simulink model "bicycle_drift_model_drive_force"  (R2016a)
settings: Solver=VariableStepAuto  StartTime=0.0  StopTime=200  MaxStep=1e-3  RelTol=1e-3
values from neighbouring files (symbols this model uses):
  a = 0.1329    [dynamics.m]    (also in setup.m; tire_test.m = 0.11372)
  b = 0.1221    [dynamics.m]    (also in setup.m; tire_test.m = 0.14328)
  C_alpha = 120000    [dynamics.m]    (also in setup.m; tire_test.m = 197)
  initial_states = [0 0 0.1]    [setup.m]
  Iz = 0.020899525    [dynamics.m]    (also in setup.m; tire_test.m = 0.025)
  L = 0.255    [dynamics.m]    (also in setup.m; tire_test.m = 0.257; veh_object2.m = obj_length)
  m = 2.622    [dynamics.m]    (also in setup.m; tire_test.m = 2.35)
  mu = 0.37    [dynamics.m]    (also in setup.m; tire_test.m = 1.31)
undefined symbols (not defined in the file): animation_update_interval, datetime, enable_CG_trace, enable_rearAxle_trace, plotAxisLimitMode, plotAxisLimits, save_anim_frames, vehicle_length, vehicle_width
libraries: simulink x2, vrlib x1
settings Model: Creator=Cyrus  LastModifiedBy=Cyrus

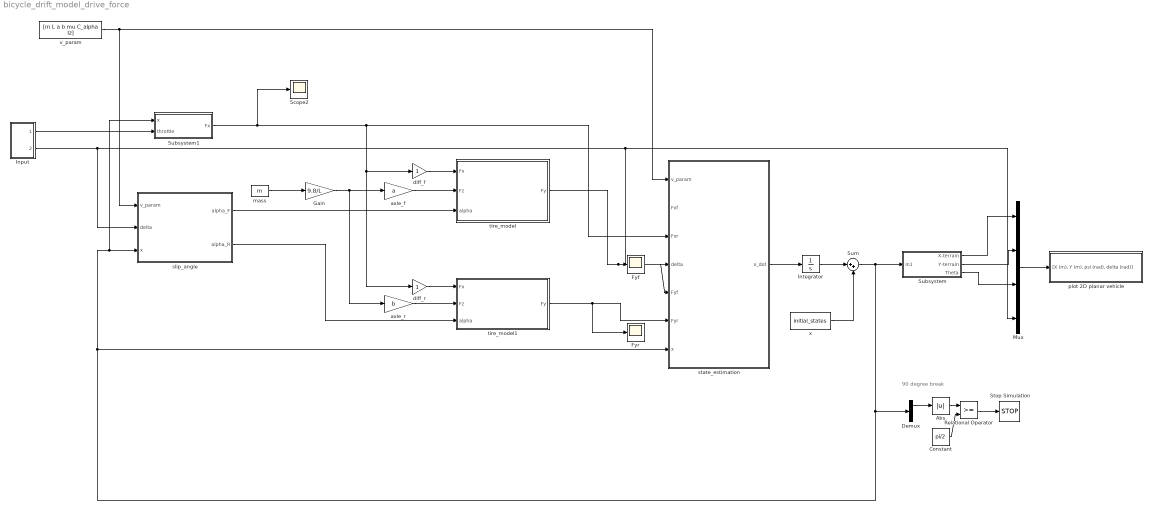
== system bicycle_drift_model_drive_force ==
  note: 90 degree break
  Abs : Abs
  Constant : Constant  Value=pi/2
  Demux : Demux  Outputs=3
  Fyf : Scope
  Fyr : Scope
  Gain : Gain  Gain=9.8/L
  Input : Subsystem
  Integrator : Integrator
  Mux : Mux
  Relational Operator : RelationalOperator  OutDataTypeStr=boolean
  Scope2 : Scope
  Stop Simulation : Stop
  Subsystem : Subsystem
  Subsystem1 : Subsystem
  Sum : Sum  Inputs=|++
  axle_f : Gain  Gain=a
  axle_r : Gain  Gain=b
  diff_f : Gain
  diff_r : Gain
  mass : Constant  Value=m
  plot 2D planar vehicle : Subsystem  mask(6DoF Animation){axisMode=plotAxisLimitMode, ax=plotAxisLimits, Ts=animation_update_interval, enable_CG_trace=enable_CG_trace, enable_rearAxle_trace=enable_rearAxle_trace, save_anim_frames=save_anim_frames, anim_frame_name_str=char(datetime('now','Format','yyyy-MM-dd_HH_mm_ss')), L=vehicle_length, W=vehicle_width}
      mask prompts: axisMode "Axis Mode (0->auto, 1->fixed, BOTH use Axes Limits below)"; ax "Axes limits [xmin xmax ymin ymax] (m):"; Ts "Time interval between updates (s):"; enable_CG_trace "Enable vehicle CG trace? (0/1)"; enable_rearAxle_trace "Enable rear axle trace? (0/1)"; save_anim_frames "Save animaton frames? (0/1)"; anim_frame_name_str "Animation sequence name (if save frames==1)"; L "Vehicle length (m)"; W "Vehicle width (m)"
      mask help:
      | Create a 2D animated view of a steering vehicle model with tires.
      |
      | Marc Compere
      | CompereM@saic.com
      | created : 22 August 2002
      | modified: 28 Dec 2015
      mask init:
      | Config.axisMode=axisMode;
      | Config.ax=ax;
      | Config.Ts=Ts;
      | Config.enable_CG_trace=enable_CG_trace;
      | Config.enable_rearAxle_trace=enable_rearAxle_trace;
      | Config.save_anim_frames=save_anim_frames;
      | Config.anim_frame_name_str=anim_frame_name_str;
      | Config.L=L;
      | Config.W=W;
      mask Help:
      | <p>This block generates a 3 dimensional display of a simulation trajectory, with the craft orientation displayed during flight</p>
      | 
      | <p>There are two inputs to this block, Position and Euler.  These inputs contain more than one signal as described below.</p>
      | 
      | <p><H4>Block Vector Input - Position</H4>
      | <ul>
      | <li>X Position</li>
      | <li>Y Position</li>
      | <li>Z Position</li>
      | </ul>
      | </p>
      | 
      | <p><H4>Block Vector Input - Euler</H4>
      |     <ul>
      |     <li>Roll Attitude</li>
      |     <li>Pitch Attitude</li>
      |     <li>Yaw Attitude</li>
      |    </ul>
      |    </p>
  slip_angle : MATLAB Function  TreatAsAtomicUnit=on
  state_estimation : MATLAB Function  TreatAsAtomicUnit=on
  tire_model : Subsystem
  tire_model1 : Subsystem
  v_param : Constant  Value=[m L a b mu C_alpha Iz]
  x : Constant  Value=initial_states
  wires:
  mass/1 -> Gain/1
  axle_f/1 -> tire_model/2(Fz)
  axle_r/1 -> tire_model1/2(Fz)
  slip_angle/1(alpha_F) -> tire_model/3(alpha)
  Gain/1 -> axle_r/1, axle_f/1
  Sum/1 -> slip_angle/3(x), Subsystem1/1(x), state_estimation/7(x), Demux/1, Subsystem/1(In1)
  state_estimation/1(x_dot) -> Integrator/1
  tire_model/1(Fy) -> Fyf/1, state_estimation/5(Fyf)
  tire_model1/1(Fy) -> Fyr/1, state_estimation/6(Fyr)
  Input/1(Throttle) -> Subsystem1/2(throttle)
  Integrator/1 -> Sum/1
  x/1 -> Sum/2
  Subsystem/1(X-terrain) -> Mux/1
  Subsystem/2(Y-terrain) -> Mux/2
  Subsystem/3("Theta ") -> Mux/3
  Mux/1 -> plot 2D planar vehicle/1("[X (m), Y (m), psi (rad), delta (rad)]")
  v_param/1 -> state_estimation/1(v_param), slip_angle/1(v_param)
  slip_angle/2(alpha_R) -> tire_model1/3(alpha)
  Input/2(Steering) -> Mux/4, state_estimation/4(delta), slip_angle/2(delta)
  diff_f/1 -> tire_model/1(Fx)
  Subsystem1/1(Fx) -> diff_f/1, diff_r/1, state_estimation/3(Fxr), Scope2/1
  diff_r/1 -> tire_model1/1(Fx)
  Demux/1 -> Abs/1
  Abs/1 -> Relational Operator/1
  Constant/1 -> Relational Operator/2
  Relational Operator/1 -> Stop Simulation/1

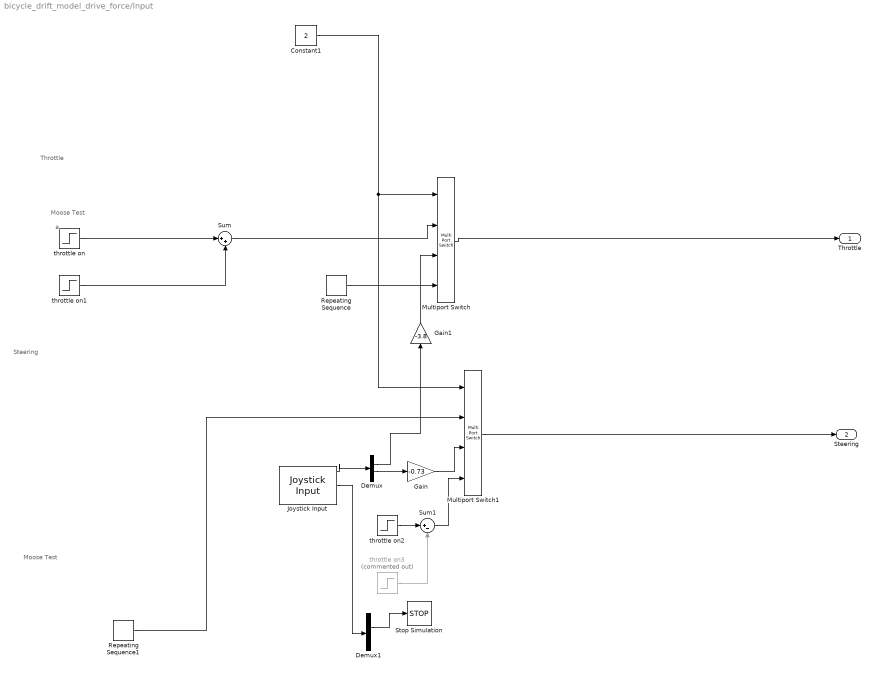
== system bicycle_drift_model_drive_force/Input ==
  note: a
  note: Steering
  note: Throttle
  note: Moose Test
  note: Moose Test
  Constant1 : Constant  Value=2
  Demux : Demux
  Demux1 : Demux  Outputs=12
  Gain : Gain  Gain=-0.73
  Gain1 : Gain  Gain=-3.8  OutMin=[0.1]
  Joystick Input : vrlib/Joystick Input  joyid=1  adjustports=on  forcefeed=off
  Multiport Switch : MultiPortSwitch
  Multiport Switch1 : MultiPortSwitch
  Repeating Sequence : simulink/Sources/Repeating Sequence  rep_seq_t=[0 2 2.1 2.5 2.6 200]  rep_seq_y=[1 1 -3.5 -3.5 0 0]
  Repeating Sequence1 : simulink/Sources/Repeating Sequence  rep_seq_t=[0 0.2 0.4 0.5 0.7 1.4 1.6 2 2.2 2.3 2.7 200]  rep_seq_y=[0 0 0.8 0.8 -0.8 -0.8 0.8 0.8 -0.8 -0.8 0 0]
  Stop Simulation : Stop
  Sum : Sum  Inputs=|++
  Sum1 : Sum  Inputs=|+-
  throttle on : Step  Time=0.2  After=2.7  SampleTime=0
  throttle on1 : Step  Time=2  After=-2.7  SampleTime=0
  throttle on2 : Step  Time=0  After=0.5  SampleTime=0
  throttle on3 : Step  Commented=on  Time=2  After=-0.8  SampleTime=0
  Throttle : Outport
  Steering : Outport  Port=2
  wires:
  Multiport Switch1/1 -> Steering/1
  Sum/1 -> Multiport Switch/2
  throttle on1/1 -> Sum/2
  throttle on/1 -> Sum/1
  Gain/1 -> Multiport Switch1/3
  Demux/3 -> Gain/1
  Joystick Input/1 -> Demux/1
  Gain1/1 -> Multiport Switch/3
  Constant1/1 -> Multiport Switch1/1, Multiport Switch/1
  Demux/2 -> Gain1/1
  Repeating Sequence/1 -> Multiport Switch/4
  Multiport Switch/1 -> Throttle/1
  throttle on2/1 -> Sum1/1
  Sum1/1 -> Multiport Switch1/4
  throttle on3/1 -> Sum1/2
  Repeating Sequence1/1 -> Multiport Switch1/2
  Joystick Input/2 -> Demux1/1
  Demux1/5 -> Stop Simulation/1

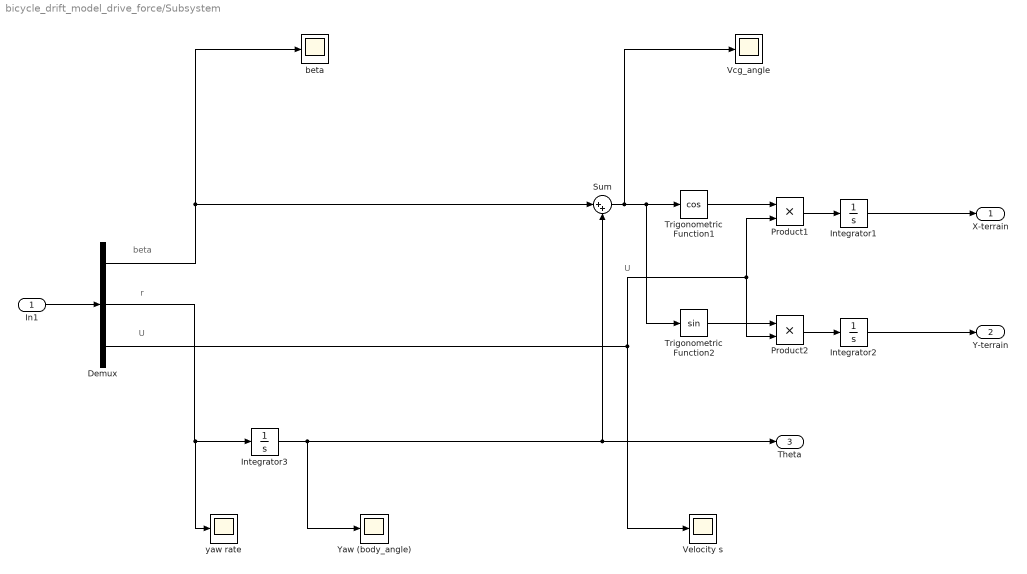
== system bicycle_drift_model_drive_force/Subsystem ==
  note: r
  note: U
  note: U
  note: beta
  In1 : Inport
  Demux : Demux  Outputs=3
  Integrator1 : Integrator
  Integrator2 : Integrator
  Integrator3 : Integrator
  Product1 : Product
  Product2 : Product
  Sum : Sum  Inputs=|++
  Trigonometric Function1 : Trigonometry  Operator=cos
  Trigonometric Function2 : Trigonometry
  Vcg_angle : Scope
  Velocity s : Scope
  Yaw (body_angle) : Scope
  beta : Scope
  yaw rate : Scope
  X-terrain : Outport
  Y-terrain : Outport  Port=2
  "Theta " : Outport  Port=3
  wires:
  In1/1 -> Demux/1
  Demux/2 -> yaw rate/1, Integrator3/1
  Demux/1 -> Sum/1, beta/1
  Trigonometric Function1/1 -> Product1/1
  Trigonometric Function2/1 -> Product2/1
  Product1/1 -> Integrator1/1
  Product2/1 -> Integrator2/1
  Integrator1/1 -> X-terrain/1
  Integrator2/1 -> Y-terrain/1
  Integrator3/1 -> "Theta "/1, Sum/2, Yaw (body_angle)/1
  Sum/1 -> Vcg_angle/1, Trigonometric Function2/1, Trigonometric Function1/1
  Demux/3 -> Product1/2, Product2/2, Velocity s/1

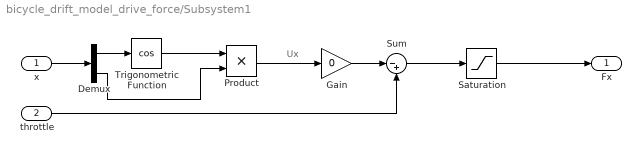
== system bicycle_drift_model_drive_force/Subsystem1 ==
  note: Ux
  x : Inport
  throttle : Inport  Port=2
  Demux : Demux  Outputs=3
  Gain : Gain  Gain=0
  Product : Product
  Saturation : Saturate  UpperLimit=mu*m*9.8*b/L  LowerLimit=-mu*m*9.8*b/L
  Sum : Sum  Inputs=|-+
  Trigonometric Function : Trigonometry  Operator=cos
  Fx : Outport
  wires:
  x/1 -> Demux/1
  Demux/3 -> Product/2
  Demux/1 -> Trigonometric Function/1
  Trigonometric Function/1 -> Product/1
  Product/1 -> Gain/1
  Gain/1 -> Sum/1
  throttle/1 -> Sum/2
  Sum/1 -> Saturation/1
  Saturation/1 -> Fx/1

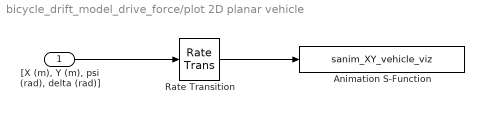
== system bicycle_drift_model_drive_force/plot 2D planar vehicle ==
  "[X (m), Y (m), psi (rad), delta (rad)]" : Inport
  Animation S-Function : S-Function  FunctionName=sanim_XY_vehicle_viz  Parameters=Config  SFunctionDeploymentMode=off  EnableBusSupport=off
  Rate Transition : RateTransition  Integrity=off
  wires:
  "[X (m), Y (m), psi (rad), delta (rad)]"/1 -> Rate Transition/1
  Rate Transition/1 -> Animation S-Function/1

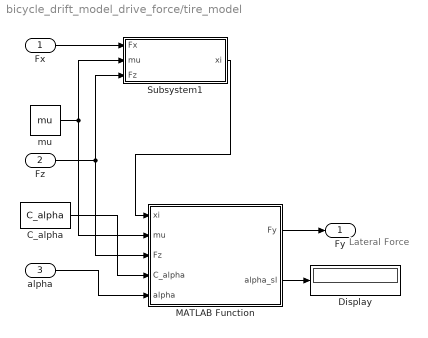
== system bicycle_drift_model_drive_force/tire_model ==
  note: Lateral Force
  Fx : Inport
  Fz : Inport  Port=2
  alpha : Inport  Port=3
  C_alpha : Constant  Value=C_alpha
  Display : Display
  MATLAB Function : MATLAB Function  TreatAsAtomicUnit=on
  Subsystem1 : Subsystem
  mu : Constant  Value=mu
  Fy : Outport
  wires:
  mu/1 -> Subsystem1/2(mu), MATLAB Function/2(mu)
  Fz/1 -> Subsystem1/3(Fz), MATLAB Function/3(Fz)
  C_alpha/1 -> MATLAB Function/4(C_alpha)
  alpha/1 -> MATLAB Function/5(alpha)
  MATLAB Function/1(Fy) -> Fy/1
  MATLAB Function/2(alpha_sl) -> Display/1
  Fx/1 -> Subsystem1/1(Fx)
  Subsystem1/1(xi) -> MATLAB Function/1(xi)

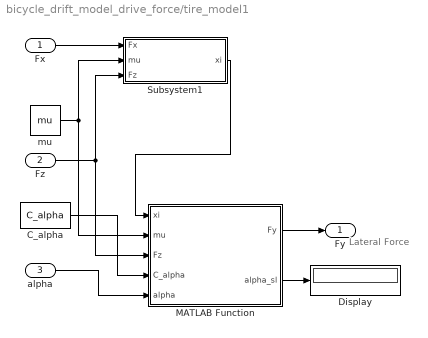
== system bicycle_drift_model_drive_force/tire_model1 ==
  note: Lateral Force
  Fx : Inport
  Fz : Inport  Port=2
  alpha : Inport  Port=3
  C_alpha : Constant  Value=C_alpha
  Display : Display
  MATLAB Function : MATLAB Function  TreatAsAtomicUnit=on
  Subsystem1 : Subsystem
  mu : Constant  Value=mu
  Fy : Outport
  wires:
  mu/1 -> Subsystem1/2(mu), MATLAB Function/2(mu)
  Fz/1 -> Subsystem1/3(Fz), MATLAB Function/3(Fz)
  C_alpha/1 -> MATLAB Function/4(C_alpha)
  alpha/1 -> MATLAB Function/5(alpha)
  MATLAB Function/1(Fy) -> Fy/1
  MATLAB Function/2(alpha_sl) -> Display/1
  Fx/1 -> Subsystem1/1(Fx)
  Subsystem1/1(xi) -> MATLAB Function/1(xi)

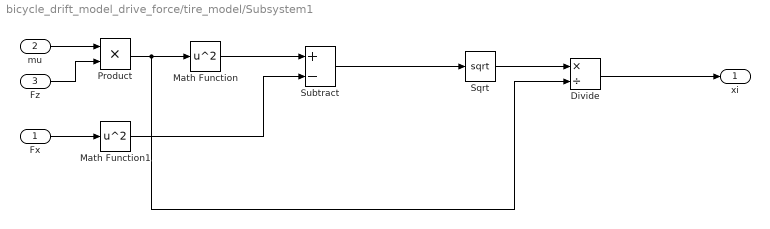
== system bicycle_drift_model_drive_force/tire_model/Subsystem1 ==
  Fx : Inport
  mu : Inport  Port=2
  Fz : Inport  Port=3
  Divide : Product  Inputs=*/
  Math Function : Math  Operator=square  SaturateOnIntegerOverflow=on
  Math Function1 : Math  Operator=square  SaturateOnIntegerOverflow=on
  Product : Product
  Sqrt : Sqrt  SaturateOnIntegerOverflow=on
  Subtract : Sum  Inputs=+-
  xi : Outport
  wires:
  mu/1 -> Product/1
  Fz/1 -> Product/2
  Product/1 -> Divide/2, Math Function/1
  Fx/1 -> Math Function1/1
  Math Function/1 -> Subtract/1
  Subtract/1 -> Sqrt/1
  Divide/1 -> xi/1
  Sqrt/1 -> Divide/1
  Math Function1/1 -> Subtract/2

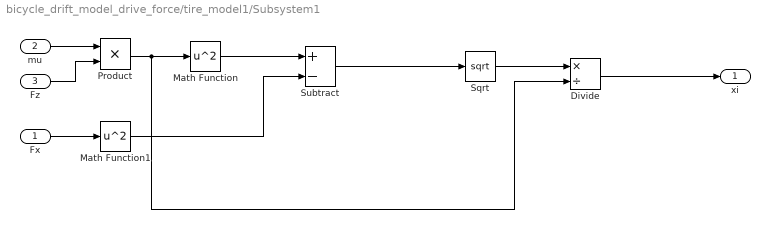
== system bicycle_drift_model_drive_force/tire_model1/Subsystem1 ==
  Fx : Inport
  mu : Inport  Port=2
  Fz : Inport  Port=3
  Divide : Product  Inputs=*/
  Math Function : Math  Operator=square  SaturateOnIntegerOverflow=on
  Math Function1 : Math  Operator=square  SaturateOnIntegerOverflow=on
  Product : Product
  Sqrt : Sqrt  SaturateOnIntegerOverflow=on
  Subtract : Sum  Inputs=+-
  xi : Outport
  wires:
  mu/1 -> Product/1
  Fz/1 -> Product/2
  Product/1 -> Divide/2, Math Function/1
  Fx/1 -> Math Function1/1
  Math Function/1 -> Subtract/1
  Subtract/1 -> Sqrt/1
  Divide/1 -> xi/1
  Sqrt/1 -> Divide/1
  Math Function1/1 -> Subtract/2

== matlab function bicycle_drift_model_drive_force/state_estimation ==
  data: v_param input; Fxf input; Fxr input; delta input; Fyf input; Fyr input; x_dot output; x input
function x_dot  = fcn(v_param,Fxf,Fxr,delta,Fyf,Fyr,x)
%#codegen
m = v_param(1);
a = v_param(3);
b = v_param(4);
Iz = v_param(7);

beta = x(1);
r = x(2);
U = x(3);
Ux = x(3)*cos(beta);
Uy = x(3)*sin(beta);

% fr = 0.002*m*9.8*sign(Ux); % rolling resistance
% if Ux < 0.01
%     fr = 0;
% end
r_dot = (a*(Fyf*cos(delta)+Fxf*sin(delta))-b*Fyr)/Iz;

Ux_dot = (Fxf*cos(delta)+Fxr-Fyf*sin(delta))/m+r*Uy;
Uy_dot = ((Fyf*cos(delta)+Fxf*sin(delta))+Fyr)/m-r*Ux;
U_dot = (2*Ux*Ux_dot+2*Uy*Uy_dot)/sqrt(2*Ux.^2+2*Uy.^2);

beta_dot = Uy_dot/Ux;
% beta_dot = (Uy_dot/Ux-((Uy*Ux_dot)/Ux.^2))/(Uy.^2/Ux.^2+1);
% Fx = Fxf*cos(delta)-Fyf*sin(delta)+Fxr;
% Fy = Fyf*cos(delta)+Fxf*sin(delta)+Fyr;
% U_dot = cos(beta)*Fx/m + sin(beta)*Fy/m;
% beta_dot = -(sin(beta)*Fx)/(m*U) + (cos(beta)*Fy)/(m*U) - r;
x_dot = [beta_dot r_dot U_dot];

== matlab function bicycle_drift_model_drive_force/slip_angle ==
  data: v_param input; delta input; x input; alpha_F output; alpha_R output
function [alpha_F, alpha_R] = fcn(v_param,delta,x)
%#codegen
a = v_param(3);
b = v_param(4);

beta = x(1);
r = x(2);
Ux = x(3)*cos(beta);
Uy = x(3)*sin(beta);
    
alpha_F = atan((Uy+a*r)/Ux)-delta;
alpha_R = atan((Uy-b*r)/Ux);

% if abs(Ux) <= 0.01
%     alpha_F = beta-delta;
%     alpha_R = beta;
% end
% if Uy+a*r > 100*Ux
%         alpha_F = pi/2-delta;
% elseif Uy+a*r < -100*Ux
%         alpha_F = -pi/2-delta;
% else
%         alpha_F = atan((Uy+a*r)/Ux)-delta;
% end
% 
% if Uy-b*r > 100*Ux
%     alpha_R = pi/2;
% elseif Uy-b*r < -100*Ux
%     alpha_R = -pi/2;
% else
%     alpha_R = atan((Uy-b*r)/Ux);
% end

== matlab function bicycle_drift_model_drive_force/tire_model/MATLAB Function ==
  data: xi input; mu input; Fz input; C_alpha input; Fy output; alpha input; alpha_sl output
function [Fy, alpha_sl] = fcn(xi, mu, Fz, C_alpha, alpha)
%#codegen
    xi_mu_Fz = xi*mu*Fz;
    alpha_sl = atan(3*xi_mu_Fz/C_alpha);

    tan_alpha = tan(alpha);

    if abs(alpha) <= alpha_sl
        Fy = -C_alpha*tan_alpha+(C_alpha.^2/(3*xi_mu_Fz))*abs(tan_alpha)*tan_alpha-(C_alpha.^3/(27*xi_mu_Fz.^2))*tan_alpha.^3;
    else
        Fy = -xi_mu_Fz*sign(alpha);
    end
end

== matlab function bicycle_drift_model_drive_force/tire_model1/MATLAB Function ==
  data: xi input; mu input; Fz input; C_alpha input; Fy output; alpha input; alpha_sl output
function [Fy, alpha_sl] = fcn(xi, mu, Fz, C_alpha, alpha)
%#codegen
    xi_mu_Fz = xi*mu*Fz;
    alpha_sl = atan(3*xi_mu_Fz/C_alpha);

    tan_alpha = tan(alpha);

    if abs(alpha) <= alpha_sl
        Fy = -C_alpha*tan_alpha+(C_alpha.^2/(3*xi_mu_Fz))*abs(tan_alpha)*tan_alpha-(C_alpha.^3/(27*xi_mu_Fz.^2))*tan_alpha.^3;
    else
        Fy = -xi_mu_Fz*sign(alpha);
    end
end
